simulink model "GBM1_2022b"  (R2022b)
settings: Solver=ode23t  StartTime=0  StopTime=130  FixedStep=0.005  MaxStep=0.005  RelTol=1e-3  EnableMultiTasking=on
values from neighbouring files (symbols this model uses):
  A1 = pi * 0.25^2    (= 0.196349540849)    [wecSimInputFile.m]
  A2 = pi * 0.01^2    (= 0.000314159265359)    [wecSimInputFile.m]
  C = 0.62    [wecSimInputFile.m]
  gDamping = 0    [wecSimInputFile.m]
  gStiffness = 0    [wecSimInputFile.m]
  rhoAir = 1.2    [wecSimInputFile.m]
  simu = simulationClass()    [wecSimInputFile.m]
  thresh = 0.3    [wecSimInputFile.m]
  waves = waveClass('irregular')    [wecSimInputFile.m]
undefined symbols (not defined in the file or in its folder): body, constraint, X, Y, Z
libraries: WECSim_Lib_Body_Elements x5, sm_lib x5, cstblocks x2, nesl_utility x2, vrlib x1, WECSim_Lib_Constraints x1, WECSim_Lib_Frames x1
(part 1 of 2)
settings Model: Creator=mlawson  LastModifiedBy=dforbus
settings SolverCC: ZeroCrossControl=DisableAll  AlgebraicLoopSolver=LineSearch  AutoInsertRateTranBlk=on
settings DataIOCC: SaveFormat=Array  SaveOutput=off  SaveTime=off  ReturnWorkspaceOutputs=off
settings OptimizationCC: LifeSpan=inf  SimCompilerOptimization=on
settings DebuggingCC: UnderspecifiedInitializationDetection=Classic  MergeDetectMultiDrivingBlocksExec=none  SolverPrmCheckMsg=warning  UnconnectedInputMsg=warning  UnconnectedOutputMsg=warning  UnconnectedLineMsg=warning  AllowSymbolicDim=off  StateNameClashWarn=warning  SFUnexpectedBacktrackingDiag=warning  SFNoUnconditionalDefaultTransitionDiag=warning  SFExecutionAtInitializationDiag=none  SFMachineParentedDataDiag=warning  ArithmeticOperatorsInVariantConditions=warning
settings HardwareCC: ProdBitPerPointer=32  ProdBitPerSizeT=32  ProdBitPerPtrDiffT=32  ProdLargestAtomicFloat=None  ProdIntDivRoundTo=Undefined  ProdEndianess=Unspecified  ProdWordSize=32  ProdHWDeviceType=32-bit Generic
settings ModelReferenceCC: EnableRefExpFcnMdlSchedulingChecks=on  PropagateSignalLabelsOutOfModel=off
settings SFSimCC: SimUseLocalCustomCode=off  CustomCodeUndefinedFunction=UseInterfaceOnly
settings RTWCC: RTWUseLocalCustomCode=off
settings CodeAppCC: StateflowObjectComments=on
settings GRTTargetCC: TargetLangStandard=C89/C90 (ANSI)
settings ConfigComp: CovMetricSettings=dw  CovSaveCumulativeToWorkspaceVar=on  CovSaveSingleToWorkspaceVar=on  CovExternalEMLEnable=off  CovSFcnEnable=off
settings SimscapeCC: SimscapeNormalizeSystem=off
settings ConfigurationSet: Description=SimMechanics 2G
settings ExplorerConfigSet: InternalSimMechanicsExplorerSettings="<ExplorerConfiguration><canonicalview>default</canonicalview><TilePanel><TileInfo><Tiles Columns=\"1\" Count=\"1\" Rows=\"1\"><Column Left=\"2\" Weight=\"1\"/><Column Left=\"1335\"/><Row Top=\"2\" Weight=\"1\"/><Row Top=\"911\"/><Tile Height=\"1\" Width=\"1\" X=\"0\" Y=\"0\"/></Tiles></TileInfo><SceneInfo><SceneViewer><BGColor><R>0.60000002384185791</R><G>0.60000002384185791</G><B>0.60000002384185791</B></BGColor><Camera><Position><X>365.37645888990272</X><Y>-369.82486814446582</Y><Z>359.64809521743916</Z></Position><Center><X>-6.7351450971904585</X><Y>2.2867358426280204</Y><Z>-12.463508769654169</Z></Center><Up><X>-0.40824829046386307</X><Y>0.40824829046386307</Y><Z>0.81649658092772615</Z></Up><Left>-57.820127362122818</Left><Right>57.820127362122818</Right><Bottom>-38.308817187253304</Bottom><Top>38.308817187253304</Top></Camera></SceneViewer></SceneInfo></TilePanel></ExplorerConfiguration>"

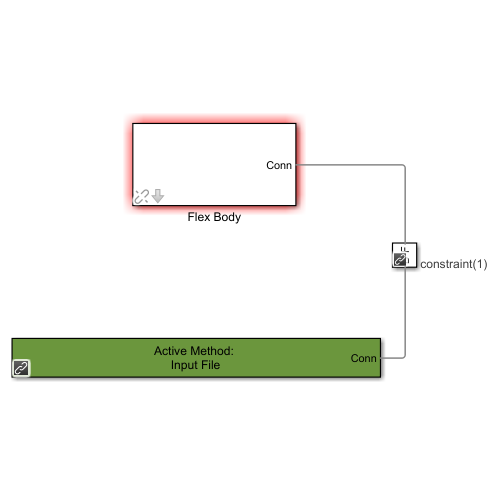
[thumbnail: Simulink's stored preview of the top-level diagram]
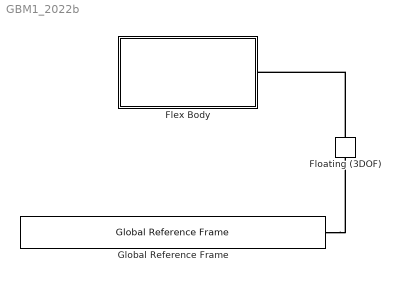
== system GBM1_2022b ==
  Flex Body : Subsystem  AncestorBlock=WECSim_Lib_Body_Elements/Flex Body  VariantControl=(default)  mask(Flex Body){body=body(1), InputFileText=Global Reference Frame option "Use Input File" is selected., h5File=hydroData/*.h5, geometryFile=geometry/*.stl, mass=0, inertia=0 0 0, nonHydro=0, nonlinearHydro=0, centerGravity=0 0 0, centerBuoyancy=0 0 0, dof=, volume=0, flex=1, displacement=0 0 0, axis=0 1 0, angle=0, option=0, cd=0 0 0, ca=0 0 0, area=0 0 0, VME=0, rgME=0 0 0, z=0 0 1}
      mask prompts: body "Body Number:"; mass "Body Mass [kg]:"; inertia "MoI [kg*m^2]:"; nonHydro "Nonhydro Body"; nonlinearHydro "Nonlinear Hydrodynamics"; centerGravity "Center of gravity [m]"; centerBuoyancy "Center of buoyancy [m]"; dof "Degrees of freedom"; volume "Displaced Volume [m^3]"; flex "Flexible Body"; displacement "Initial Linear Displacement"; axis "Initial Angular Displacement Axis"; angle "Initial Angular Displacement"; option "On/Off"; cd "Drag coefficient"; ca "Added mass coefficient"; area "Characteristic Area"; VME "Characteristic Volume"; rgME "Point of Application"; z "Z axis"
      mask help:
      | A Flex Body may contain generalized body modes that account for various bending, shear or other deformation modes. The BEM output must contain data for these additional DOFs.
      |
      | The variable name input below must be 'body(i)' where i=1,2,...
      | body(i) must be defined in the input file with the following fields:
      |
      |     .flexHydroBody = 1 (required)
      |             Float.
      |             Flag that creates a flex body. Set equal to 1 if the BEM data contains more than 6 degrees of freedom.
      |     .filename (required)
      |             String.
      |             The file path specifying the .h5 file for the body.
      |     .mass (required)
      |             Float or string.
      |             The translational interia or mass of the body in kg. If a string, the value must be 'equilibrium'. Default = [ ]
      |     .momOfIntertia (required)
      |             3x1 vector [Ixx Iyy Izz].
      |             Rotational intertia of the body in kg*m^2. Default = [ ]
      |     .geometryFile (optional)
      |             String
      |             Path to the geometry file of the body (.stl). Required for nonlinear hydrodynamics or visualization. Default = [ ]
      mask init:
      | if exist('body','var')
      |     % geometry file name
      |     h=[gcb '/Structure/Body Properties'];
      |     geomFile=body.geometryFile;
      |     set_param(h,'ExtGeomFileName',geomFile);
      |     geomType='STL';
      |     % split version e.g. '9.10.0.16028 (R2021a)' into 9, 10, 0, NaN.
      |     % cannot compare str2double('9.10') because it becomes '9.1' 
      |     ver=split(version,'.');
      |     ver=str2double(ver(1:3));
      |     if ver(1) < 9 || (ver(1) == 9 && ver(2) < 6)
      |        set_param(h,'ExtGeomFileType',geomType);
      |     end
      |     % toWorkSpace: outputs
      |     h=[gcb '/To Workspace'];
      |     responseName=['body' num2str(body.number) '_out'];
      |     set_param(h,'VariableName',responseName);
      |     % toWorkSpace: hydrostatic pressures
      |     h=[gcb '/Hydrostatic Restoring Force Calculation/Hydrostatic Restoring Force Calculation/Linear and Nonlinear Restoring Force Variant Subsystem/Nonlinear Hydrostatic Restoring Force/To Workspace1'];
      |     responseName=['body' num2str(body.number) '_hspressure_out'];
      |     set_param(h,'VariableName',responseName); 
      |     % toWorkSpace: wave pressures (nonlinear Froude-Krylov)
      |     h=[gcb '/Wave Diffraction and Excitation Force Calculation/Wave Diffraction and Excitation Force Calculation/Nonlinear FK Force Variant Subsystem/With Nonlinear FroudeKrylov Force/To Workspace'];
      |     responseName=['body' num2str(body.number) '_wavenonlinearpressure_out'];
      |     set_param(h,'VariableName',responseName);
      |     % toWorkSpace: wave pressures (linear Froude-Krylov)
      |     h=[gcb '/Wave Diffraction and Excitation Force Calculation/Wave Diffraction and Excitation Force Calculation/Nonlinear FK Force Variant Subsystem/With Nonlinear FroudeKrylov Force/To Workspace1'];
      |     responseName=['body' num2str(body.number) '_wavelinearpressure_out'];
      |     set_param(h,'VariableName',responseName);
      |     % position: GoTo 
      |     h=[gcb '/Goto'];
      |     responseName=['disp' num2str(body.number)];
      |     set_param(h,'GotoTag',responseName);
      |     % position: From
      |     h=[gcb '/From'];
      |     responseName=['disp' num2str(body.number)];
      |     set_param(h,'GotoTag',responseName);
      |     % velocity: GoTo 
      |     h=[gcb '/Goto1'];
      |     responseName=['vel' num2str(body.number)];
      |     set_param(h,'GotoTag',responseName);
      |     % velocity: From 
      |     h=[gcb '/From1'];
      |     responseName=['vel' num2str(body.number)];
      |     set_param(h,'GotoTag',responseName);
      |     % acceleration: GoTo 
      |     h=[gcb '/Goto2'];
      |     responseName=['acc' num2str(body.number)];
      |     set_param(h,'GotoTag',responseName);
      |     % acceleration: From 
      |     h=[gcb '/From2'];
      |     responseName=['acc' num2str(body.number)];
      |     set_param(h,'GotoTag',responseName);
      |     %%
      |     % Flex Body Morison Element: Off
      |     h = [gcb '/Morrison Element and Viscous Damping Force Calculation/Morison Element and Viscous Damping Force Calculation/Morison Element Variant Subsystem/Morison Element Off'];
      |     responseName = ['sv_b' num2str(body.number) '_MEOff'];
      |     set_param(h,'VariantControl',responseName);
      |     %%
      |     % Flex Body Morison Element: On
      |     h = [gcb '/Morrison Element and Viscous Damping Force Calculation/Morison Element and Viscous Damping Force Calculation/Morison Element Variant Subsystem/Morison Element On'];
      |     responseName = ['sv_b' num2str(body.number) '_MEOn'];
      |     set_param(h,'VariantControl',responseName);
      |     %%
      |     % Flex Body Nonlinear FroudeKrylov Force: Off
      |     h = [gcb '/Wave Diffraction and Excitation Force Calculation/Wave Diffraction and Excitation Force Calculation/Nonlinear FK Force Variant Subsystem/No Nonlinear FroudeKrylov Force'];
      |     responseName = ['sv_b' num2str(body.number) '_linearHydro'];
      |     set_param(h,'VariantControl',responseName);
      |     %%
      |     % Flex Body Nonlinear FroudeKrylov Force: On
      |     h = [gcb '/Wave Diffraction and Excitation Force Calculation/Wave Diffraction and Excitation Force Calculation/Nonlinear FK Force Variant Subsystem/With Nonlinear FroudeKrylov Force'];
      |     responseName = ['sv_b' num2str(body.number) '_nonlinearHydro'];
      |     set_param(h,'VariantControl',responseName);
      |     %%
      |     % Flex Body Nonlinear Restoring: Off
      |     h = [gcb '/Hydrostatic Restoring Force Calculation/Hydrostatic Restoring Force Calculation/Linear and Nonlinear Restoring Force Variant Subsystem/Linear Hydrostatic Restoring Force'];
      |     responseName = ['sv_b' num2str(body.number) '_linearHydro'];
      |     set_param(h,'VariantControl',responseName);
      |     %%
      |     % Flex Body Nonlinear Restoring: On
      |     h = [gcb '/Hydrostatic Restoring Force Calculation/Hydrostatic Restoring Force Calculation/Linear and Nonlinear Restoring Force Variant Subsystem/Nonlinear Hydrostatic Restoring Force'];
      |     responseName = ['sv_b' num2str(body.number) '_nonlinearHydro'];
      |     set_param(h,'VariantControl',responseName);
      |     %%
      |     % Flex Body Nonlinear FroudeKrylov or Restoring: Instantaneous Free Surface
      |     h = [gcb '/Nonlinear Wave Elevation/Linear or Instantaneous Free Surface/Instantaneous Water Free Surface'];
      |     responseName = ['sv_b' num2str(body.number) '_instFS'];
      |     set_param(h,'VariantControl',responseName);
      |     %%
      |     % Flex Body Nonlinear FroudeKrylov or Restoring: Mean Free Surface
      |     h = [gcb '/Nonlinear Wave Elevation/Linear or Instantaneous Free Surface/Mean Water Free Surface'];
      |     responseName = ['sv_b' num2str(body.number) '_meanFS'];
      |     set_param(h,'VariantControl',responseName);
      |     %%
      | end
      settings: LibrarySourceBlock=WECSim_Lib_Body_Elements/Flex Body
      mask Help:
      | A Flex Body may contain generalized body modes that account for various bending, shear or other deformation modes. The BEM output must contain data for these additional DOFs.
      | 
      | The variable name input below must be 'body(i)' where i=1,2,...
      | body(i) must be defined in the input file with the following fields:
      | 
      |     .flexHydroBody = 1 (required)
      |             Float.
      |             Flag that creates a flex body. Set equal to 1 if the BEM data contains more than 6 degrees of freedom.
      |     .filename (required)
      |             String.
      |             The file path specifying the .h5 file for the body.
      |     .mass (required)
      |             Float or string.
      |             The translational interia or mass of the body in kg. If a string, the value must be 'equilibrium'. Default = [ ]
      |     .momOfIntertia (required)
      |             3x1 vector [Ixx Iyy Izz].
      |             Rotational intertia of the body in kg*m^2. Default = [ ]
      |     .geometryFile (optional)
      |             String
      |             Path to the geometry file of the body (.stl). Required for nonlinear hydrodynamics or visualization. Default = [ ]
      mask TypeOptions nonHydro: 0 | 1 | 2
      mask Callback nonHydro: bodyClassCallback(gcbh)
      mask TypeOptions nonlinearHydro: 0 | 1 | 2
      mask TypeOptions flex: 0 | 1
      mask TypeOptions option: 0 | 1 | 2
      mask Callback option: bodyClassCallback(gcbh)
      mask DialogControl CustomParameterGroup Prompt: Custom Parameters
      mask DialogControl std_opts Prompt: Standard Options
      mask DialogControl H5button Prompt: Select .h5 File
      mask DialogControl H5button Callback: h5ButtonCallback(gcbh)
      mask DialogControl STLbutton Prompt: Select .stl File
      mask DialogControl STLbutton Callback: stlButtonCallback(gcbh)
      mask DialogControl inertia Tooltip: Moment of Inertia
      mask DialogControl initial Prompt: Initial Displacement
      mask DialogControl morisonElement Prompt: Morison Element
      mask DialogControl rgME Tooltip: The vector from the body COG to point of application for the Morison Element
      mask DialogControl z Tooltip: The unit normal vector center axis of the Morison Element
  Floating (3DOF) : WECSim_Lib_Constraints/Floating (3DOF)  constraint=constraint(1)  loc="0  0  0"  displacement=0 0 0  y=0 1 0  z=0 0 1  upperLimitSpecify=off  upperLimitBound=0  upperLimitTransitionRegionWidth=0  upperLimitStiffness=0  upperLimitDamping=0  lowerLimitSpecify=off  lowerLimitBound=0  lowerLimitTransitionRegionWidth=0  lowerLimitStiffness=0  lowerLimitDamping=0
      settings: AttributesFormatString=%<constraint>
  Global Reference Frame : WECSim_Lib_Frames/Global Reference Frame  waves=waves  simu=simu  InputMethod=Input File  InputFile=wecSimInputFile.m  mode=normal  explorer=off  solver=ode4  startTime=0  rampTime=100  endTime=400  dt=0.1  cicEndTime=60  stateSpace=0  WaveClass=regular  height=2.5  period=8  elevationFile=NOT DEFINED  spectrumFile=NOT DEFINED  direction=0  spread=1  spectrumType=NOT DEFINED  phaseSeed=0  option=EqualEnergy
  connections:
  Global Reference Frame/RConn1 -- Floating (3DOF)/LConn1
  Floating (3DOF)/RConn1 -- Flex Body/RConn1

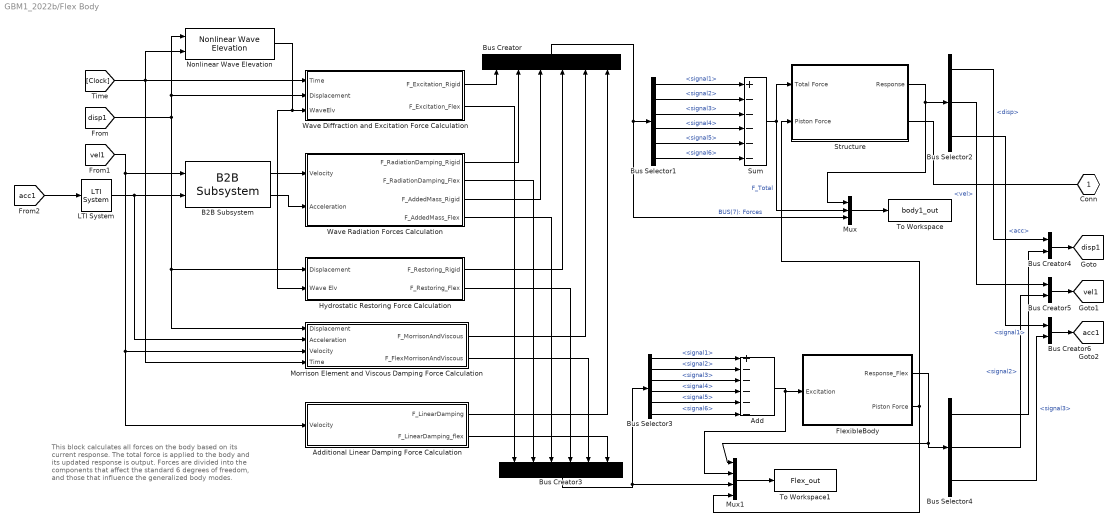
== system GBM1_2022b/Flex Body ==
  note: This block calculates all forces on the body based on its current response. The total force is applied to the body and its updated response is output.
      |
      | Forces are divided into the components that affect the standard 6 degrees of freedom, and those that influence the generalized body modes.
  Add : Sum  Inputs=+-----
  Additional Linear Damping Force Calculation : Subsystem
  B2B Subsystem : WECSim_Lib_Body_Elements/Rigid Body/Hydrodynamic Body/B2B Subsystem  SystemSampleTime=-1  VariantActivationTime=update diagram  Latency=0  AutoFrameSizeCalculation=off
  Bus Creator : BusCreator  Inputs=6
  Bus Creator3 : BusCreator  Inputs=6
  Bus Creator4 : BusCreator  Inputs=2
  Bus Creator5 : BusCreator  Inputs=2
  Bus Creator6 : BusCreator  Inputs=2
  Bus Selector1 : BusSelector  OutputSignals=signal1,signal2,signal3,signal4,signal5,signal6
  Bus Selector2 : BusSelector  OutputSignals=disp,vel,acc
  Bus Selector3 : BusSelector  OutputSignals=signal1,signal2,signal3,signal4,signal5,signal6
  Bus Selector4 : BusSelector  OutputSignals=signal1,signal2,signal3
  FlexibleBody : Subsystem
  Hydrostatic Restoring Force Calculation : Subsystem
  LTI System : cstblocks/LTI System  sys=LPF50  IC=[]
  Morrison Element and Viscous Damping Force Calculation : Subsystem
  Mux : Mux  Inputs=3
  Mux1 : Mux
  Nonlinear Wave Elevation : WECSim_Lib_Body_Elements/Rigid Body/Hydrodynamic Body/Nonlinear Wave Elevation  SystemSampleTime=simu.nonlinearDt  VariantActivationTime=update diagram  Latency=0  AutoFrameSizeCalculation=off
  Structure : Subsystem
  Sum : Sum  Inputs=+-----
  To Workspace : ToWorkspace  VariableName=body1_out  SaveFormat=Structure With Time  SampleTime=simu.dtOut
  To Workspace1 : ToWorkspace  VariableName=Flex_out  SaveFormat=Structure With Time  SampleTime=simu.dtOut
  Wave Diffraction and Excitation Force Calculation : Subsystem
  Wave Radiation Forces Calculation : Subsystem
  Conn : PMIOPort  Side=Right
  tag scope: acc1=global, disp1=global, vel1=global
  wires:
  LTI System/1 -> Morrison Element and Viscous Damping Force Calculation/2(Acceleration), B2B Subsystem/2
  [acc1] -> LTI System/1
  Morrison Element and Viscous Damping Force Calculation/1(F_MorrisonAndViscous) -> Bus Creator/5
  Hydrostatic Restoring Force Calculation/2(F_Restoring_Flex) -> Bus Creator3/4
  Bus Selector2/3 -> Bus Creator6/1  "<acc>"
  Bus Selector2/2 -> Bus Creator5/1  "<vel>"
  Bus Creator6/1 -> [acc1]
  Bus Creator5/1 -> [vel1]
  Bus Creator4/1 -> [disp1]
  Bus Selector2/1 -> Bus Creator4/1  "<disp>"
  Bus Selector3/6 -> Add/6  "<signal6>"
  Additional Linear Damping Force Calculation/2(F_LinearDamping_flex) -> Bus Creator3/6
  Bus Selector3/5 -> Add/5  "<signal5>"
  Morrison Element and Viscous Damping Force Calculation/2("F_FlexMorrisonAndViscous ") -> Bus Creator3/5
  Additional Linear Damping Force Calculation/1(F_LinearDamping) -> Bus Creator/6
  Bus Selector4/3 -> Bus Creator6/2  "<signal3>"
  Bus Selector4/2 -> Bus Creator5/2  "<signal2>"
  Bus Selector4/1 -> Bus Creator4/2  "<signal1>"
  FlexibleBody/1(Response_Flex) -> Mux1/1, Bus Selector4/1
  Add/1 -> FlexibleBody/1(Excitation), Mux1/2
  Bus Selector3/4 -> Add/4  "<signal4>"
  Bus Selector3/3 -> Add/3  "<signal3>"
  Bus Selector3/2 -> Add/2  "<signal2>"
  Bus Selector3/1 -> Add/1  "<signal1>"
  Bus Creator3/1 -> Mux1/3, Bus Selector3/1
  Wave Radiation Forces Calculation/4(F_AddedMass_Flex) -> Bus Creator3/3
  Wave Radiation Forces Calculation/2(F_RadiationDamping_Flex) -> Bus Creator3/2
  Wave Diffraction and Excitation Force Calculation/2(F_Excitation_Flex) -> Bus Creator3/1
  Mux1/1 -> To Workspace1/1
  [Clock] -> Wave Diffraction and Excitation Force Calculation/1(Time), Morrison Element and Viscous Damping Force Calculation/4(Time), Nonlinear Wave Elevation/2
  Wave Radiation Forces Calculation/3(F_AddedMass_Rigid) -> Bus Creator/3
  Wave Diffraction and Excitation Force Calculation/1(F_Excitation_Rigid) -> Bus Creator/1
  Wave Radiation Forces Calculation/1(F_RadiationDamping_Rigid) -> Bus Creator/2
  Hydrostatic Restoring Force Calculation/1(F_Restoring_Rigid) -> Bus Creator/4
  Nonlinear Wave Elevation/1 -> Wave Diffraction and Excitation Force Calculation/3(WaveElv), Hydrostatic Restoring Force Calculation/2(Wave Elv)
  [disp1] -> Hydrostatic Restoring Force Calculation/1(Displacement), Morrison Element and Viscous Damping Force Calculation/1(Displacement), Wave Diffraction and Excitation Force Calculation/2(Displacement), Nonlinear Wave Elevation/1
  B2B Subsystem/1 -> Wave Radiation Forces Calculation/1(Velocity)
  B2B Subsystem/2 -> Wave Radiation Forces Calculation/2(Acceleration)
  [vel1] -> B2B Subsystem/1, Morrison Element and Viscous Damping Force Calculation/3(Velocity), Additional Linear Damping Force Calculation/1(Velocity)
  Bus Selector1/6 -> Sum/6  "<signal6>"
  Bus Selector1/1 -> Sum/1  "<signal1>"
  Bus Selector1/2 -> Sum/2  "<signal2>"
  Bus Selector1/5 -> Sum/5  "<signal5>"
  Bus Selector1/3 -> Sum/3  "<signal3>"
  Bus Selector1/4 -> Sum/4  "<signal4>"
  Mux/1 -> To Workspace/1
  Sum/1 -> Structure/1(Total Force), Mux/2  "F_Total"
  Structure/1(Response) -> Bus Selector2/1, Mux/1
  Bus Creator/1 -> Bus Selector1/1, Mux/3  "BUS(7): Forces"
  FlexibleBody/2(Piston Force) -> Structure/2(Piston Force), Mux1/4
  connections:
  Conn/RConn1 -- Structure/RConn1

== system GBM1_2022b/Flex Body/Additional Linear Damping Force Calculation ==
  Velocity : Inport
  Additional Linear Damping Force Calculation : WECSim_Lib_Body_Elements/Rigid Body/Hydrodynamic Body/Additional Linear Damping Force Calculation  SystemSampleTime=-1  VariantActivationTime=update diagram  Latency=0  AutoFrameSizeCalculation=off
  Selector : Selector  InputPortWidth=body.dof  IndexOptions=Index vector (dialog)  Indices=[1:6]  OutputSizes=1
  Selector1 : Selector  InputPortWidth=body.dof  IndexOptions=Index vector (dialog)  Indices=[7:body.dofEnd]  OutputSizes=1
  F_LinearDamping : Outport  PortDimensions=6
  F_LinearDamping_flex : Outport  Port=2  PortDimensions=body.gbmDOF
  wires:
  Additional Linear Damping Force Calculation/1 -> Selector1/1, Selector/1
  Velocity/1 -> Additional Linear Damping Force Calculation/1  "v"
  Selector1/1 -> F_LinearDamping_flex/1
  Selector/1 -> F_LinearDamping/1

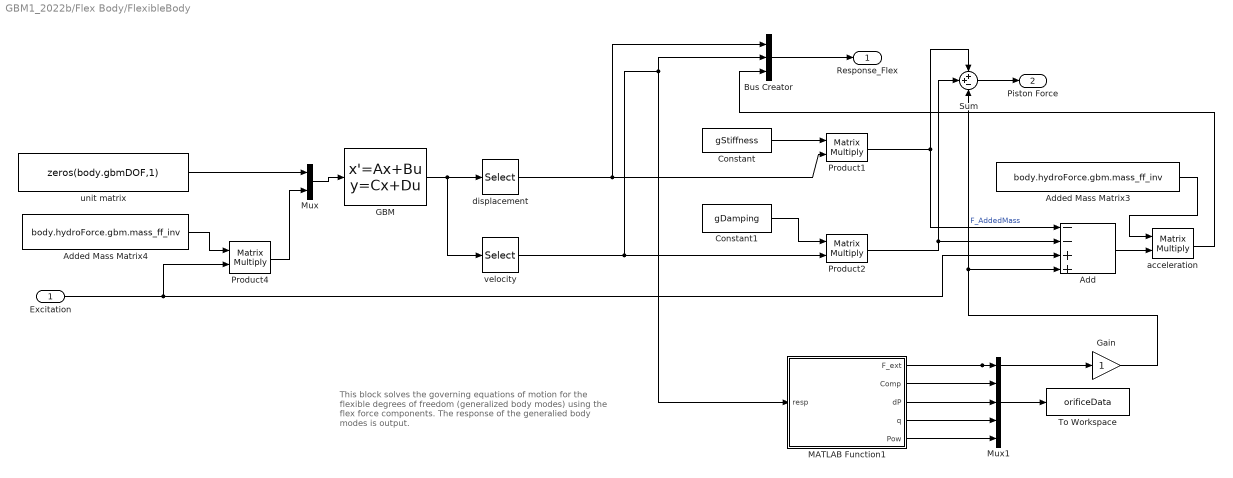
== system GBM1_2022b/Flex Body/FlexibleBody ==
  note: This block solves the governing equations of motion for the flexible degrees of freedom (generalized body modes) using the flex force components. The response of the generalied body modes is output.
  Excitation : Inport
  Add : Sum  Inputs=--++
  Added Mass Matrix3 : Constant  Value=body.hydroForce.gbm.mass_ff_inv
  Added Mass Matrix4 : Constant  Value=body.hydroForce.gbm.mass_ff_inv
  Bus Creator : BusCreator  Inputs=3
  Constant : Constant  Value=gStiffness
  Constant1 : Constant  Value=gDamping
  GBM : StateSpace  A=body.hydroForce.gbm.state_space.A  B=body.hydroForce.gbm.state_space.B  C=body.hydroForce.gbm.state_space.C  D=body.hydroForce.gbm.state_space.D  InitialCondition=0
  Gain : Gain
  MATLAB Function1 : MATLAB Function  TreatAsAtomicUnit=on
  Mux : Mux  Inputs=2
  Mux1 : Mux  Inputs=5
  Product1 : Product  Multiplication=Matrix(*)
  Product2 : Product  Multiplication=Matrix(*)
  Product4 : Product  Multiplication=Matrix(*)
  Sum : Sum  Inputs=++-
  To Workspace : ToWorkspace  VariableName=orificeData  SaveFormat=Structure With Time  SampleTime=-1
  acceleration : Product  Multiplication=Matrix(*)
  displacement : Selector  InputPortWidth=body.gbmDOF*2  IndexOptions=Index vector (dialog)  Indices=[1:body.gbmDOF]  OutputSizes=1
  unit matrix : Constant  Value=zeros(body.gbmDOF,1)
  velocity : Selector  InputPortWidth=2*body.gbmDOF  IndexOptions=Index vector (dialog)  Indices=[body.gbmDOF+1:2*body.gbmDOF]  OutputSizes=1
  Response_Flex : Outport
  Piston Force : Outport  Port=2
  wires:
  acceleration/1 -> Bus Creator/3
  Bus Creator/1 -> Response_Flex/1
  Mux/1 -> GBM/1
  Product4/1 -> Mux/2
  Added Mass Matrix4/1 -> Product4/1
  unit matrix/1 -> Mux/1
  Add/1 -> acceleration/2
  Added Mass Matrix3/1 -> acceleration/1
  Product1/1 -> Add/1, Sum/1  "F_AddedMass"
  Constant1/1 -> Product2/1
  Constant/1 -> Product1/1
  GBM/1 -> velocity/1, displacement/1
  Product2/1 -> Sum/2, Add/2
  Sum/1 -> Piston Force/1
  MATLAB Function1/1(F_ext) -> Mux1/1, Gain/1
  Mux1/1 -> To Workspace/1
  MATLAB Function1/2(Comp) -> Mux1/2
  MATLAB Function1/3(dP) -> Mux1/3
  MATLAB Function1/4(q) -> Mux1/4
  MATLAB Function1/5(Pow) -> Mux1/5
  velocity/1 -> MATLAB Function1/1(resp), Bus Creator/2, Product2/2
  displacement/1 -> Bus Creator/1, Product1/2
  Excitation/1 -> Add/3, Product4/2
  Gain/1 -> Add/4, Sum/3

== system GBM1_2022b/Flex Body/Hydrostatic Restoring Force Calculation ==
  note: Do not link the `Hydrostatic Restoring Force Calculation`
      | to the rigid body block, this will break the Flex Body block.
  Displacement : Inport
  Wave Elv : Inport  Port=2
  Hydrostatic Restoring Force Calculation : Subsystem
  Selector : Selector  InputPortWidth=body.dof  IndexOptions=Index vector (dialog)  Indices=[1:6]  OutputSizes=1
  Selector1 : Selector  InputPortWidth=body.dof  IndexOptions=Index vector (dialog)  Indices=[7:body.dofEnd]  OutputSizes=1
  F_Restoring_Rigid : Outport  PortDimensions=6
  F_Restoring_Flex : Outport  Port=2  PortDimensions=body.gbmDOF
  wires:
  Wave Elv/1 -> Hydrostatic Restoring Force Calculation/2(Wave Elv)
  Displacement/1 -> Hydrostatic Restoring Force Calculation/1(Displacement)  "x"
  Selector1/1 -> F_Restoring_Flex/1
  Selector/1 -> F_Restoring_Rigid/1
  Hydrostatic Restoring Force Calculation/1(F_Restoring) -> Selector/1, Selector1/1  "F_Restoring"

== system GBM1_2022b/Flex Body/Morrison Element and Viscous Damping Force Calculation ==
  Displacement : Inport
  Acceleration : Inport  Port=2
  Velocity : Inport  Port=3
  Time : Inport  Port=4
  Morison Element and Viscous Damping Force Calculation : Subsystem  AncestorBlock=WECSim_Lib_Body_Elements/Rigid Body/Hydrodynamic Body/Morison Element and Viscous Damping Force Calculation
      settings: LibrarySourceBlock=WECSim_Lib_Body_Elements/Rigid Body/Hydrodynamic Body/Morison Element and Viscous Damping Force Calculation
  Selector : Selector  InputPortWidth=body.dof  IndexOptions=Index vector (dialog)  Indices=[1:6]  OutputSizes=1
  Selector1 : Selector  InputPortWidth=body.dof  IndexOptions=Index vector (dialog)  Indices=[7:body.dofEnd]  OutputSizes=1
  F_MorrisonAndViscous : Outport  PortDimensions=6
  "F_FlexMorrisonAndViscous " : Outport  Port=2  PortDimensions=body.gbmDOF
  wires:
  Selector1/1 -> "F_FlexMorrisonAndViscous "/1
  Selector/1 -> F_MorrisonAndViscous/1
  Morison Element and Viscous Damping Force Calculation/1(F_MorisonAndViscous) -> Selector/1, Selector1/1
  Velocity/1 -> Morison Element and Viscous Damping Force Calculation/3(Velocity)
  Displacement/1 -> Morison Element and Viscous Damping Force Calculation/1(Displacement)
  Time/1 -> Morison Element and Viscous Damping Force Calculation/4(Time)
  Acceleration/1 -> Morison Element and Viscous Damping Force Calculation/2(Acceleration)

== system GBM1_2022b/Flex Body/Structure ==
  note: Apply the total force to the body and calculate its response relative to the global reference frame.
      |
      | Output force to apply to another body.
  Total Force : Inport
  Piston Force : Inport  Port=2
  Body Properties : sm_lib/Body Elements/File Solid  ExtGeomFileName=../geometry/float.stl  UnitType=Custom  ExtGeomFileUnits=m  StepReaderType=HEX  ExportConvexHullGeometry=off  InertiaType=Custom  Mass=body.mass  MassUnits=kg  CenterOfMass=[0 0 0]  CenterOfMassUnits=m  MomentsOfInertia=body.inertia  MomentsOfInertiaUnits=kg*m^2  ProductsOfInertia=[0 0 0]  ProductsOfInertiaUnits=kg*m^2  BasedOnType=Density  Density=1000  DensityUnits=kg/(m^3)  DoExposeReferenceFrame=on  SerializedFrames=<Frames/>  GraphicType=FromGeometry  MarkerShape=Sphere  MarkerSize=10  MarkerSizeUnits=m  GraphicVisPropType=SimpleVisualProperties  GraphicDiffuseColor=body.viz.color  GraphicSpecularColor=[0.5 0.5 0.5 1.0]  GraphicAmbientColor=[0.15 0.15 0.15 1.0]  GraphicEmissiveColor=[0.0 0.0 0.0 1.0]  GraphicShininess=75  GraphicOpacity=body.viz.opacity
  Demux : Demux  Outputs=3
  External Force and Torque : sm_lib/Forces and Torques/External Force and Torque  ForceResolutionFrame=World  EnableForceX=off  EnableForceY=off  EnableForceZ=off  EnableForce=on  TorqueResolutionFrame=World  EnableTorqueX=off  EnableTorqueY=off  EnableTorqueZ=off  EnableTorque=on
  Motion Sensor : WECSim_Lib_Body_Elements/Rigid Body/Hydrodynamic Body/Structure/Motion Sensor  SystemSampleTime=-1  VariantActivationTime=update diagram  Latency=0  AutoFrameSizeCalculation=off
  Mux : Mux  Inputs=3
  Rigid Transform (Setup CG) : sm_lib/Frames and Transforms/Rigid Transform  TranslationMethod=Cartesian  TranslationStandardOffset=0  TranslationLengthUnit=m  TranslationStandardAxis=+Z  TranslationCartesianOffset=body.centerGravity  TranslationROffset=0  TranslationROffsetUnits=m  TranslationZOffset=0  TranslationZOffsetUnits=m  TranslationThetaOffset=0  TranslationThetaOffsetUnits=deg  RotationMethod=None  RotationAngleUnits=rad  RotationStandardAxis=+Y  RotationAngle=0.05  RotationArbitraryAxis=[0.57735026918962584 0.57735026918962584 0.57735026918962584]  FollAlignAxisA=+X  BaseAlignAxisA=+Y  FollAlignAxisB=+Y  BaseAlignAxisB=+Z  RotationSequenceAxes=FollowerAxes  RotationSequence=XYX  RotationSequenceAngles=[0 0 0]  RotationSequenceAnglesUnits=deg  RotationMatrix=[1 0 0; 0 1 0; 0 0 1]  Quaternion=[1 0 0 0]
  Rigid Transform (Setup Initial Disp) : sm_lib/Frames and Transforms/Rigid Transform  TranslationMethod=Cartesian  TranslationStandardOffset=0  TranslationLengthUnit=m  TranslationStandardAxis=+Z  TranslationCartesianOffset=body.initial.displacement  TranslationROffset=0  TranslationROffsetUnits=m  TranslationZOffset=0  TranslationZOffsetUnits=m  TranslationThetaOffset=0  TranslationThetaOffsetUnits=deg  RotationMethod=ArbitraryAxis  RotationAngleUnits=rad  RotationStandardAxis=+Y  RotationAngle=body.initial.angle  RotationArbitraryAxis=body.initial.axis  FollAlignAxisA=+X  BaseAlignAxisA=+Y  FollAlignAxisB=+Y  BaseAlignAxisB=+Z  RotationSequenceAxes=FollowerAxes  RotationSequence=XYX  RotationSequenceAngles=[0 0 0]  RotationSequenceAnglesUnits=deg  RotationMatrix=[1 0 0; 0 1 0; 0 0 1]  Quaternion=[1 0 0 0]
  Selector : Selector  InputPortWidth=6  IndexOptions=Index vector (dialog)  Indices=[1:3]  OutputSizes=1
  Selector1 : Selector  InputPortWidth=6  IndexOptions=Index vector (dialog)  Indices=[4:6]  OutputSizes=1
  Simulink-PS Converter1 : nesl_utility/Simulink-PS Converter  PhysicalDomain=network_engine_domain  SubClassName=ps_input  LeftPortType=input  RightPortType=output  PseudoPeriodic=off  Frequencies=[]  NoiseDistribution=none  NoiseParameters=[]  Unit=1  AffineConversion=off  FilteringAndDerivatives=zero  SimscapeFilterOrder=1  InputFilterTimeConstant=0.001  UdotUserProvided=1
  Simulink-PS Converter2 : nesl_utility/Simulink-PS Converter  PhysicalDomain=network_engine_domain  SubClassName=ps_input  LeftPortType=input  RightPortType=output  PseudoPeriodic=off  Frequencies=[]  NoiseDistribution=none  NoiseParameters=[]  Unit=1  AffineConversion=off  FilteringAndDerivatives=zero  SimscapeFilterOrder=1  InputFilterTimeConstant=0.001  UdotUserProvided=1
  Sum : Sum  Inputs=++|
  World Frame : sm_lib/Frames and Transforms/World Frame
  Conn Free Surface : PMIOPort  Side=Right
  Response : Outport
  wires:
  Motion Sensor/1 -> Response/1
  Selector1/1 -> Simulink-PS Converter2/1
  Total Force/1 -> Selector/1, Selector1/1
  Selector/1 -> Demux/1
  Mux/1 -> Simulink-PS Converter1/1
  Demux/3 -> Sum/2
  Sum/1 -> Mux/3
  Piston Force/1 -> Sum/1
  Demux/2 -> Mux/2
  Demux/1 -> Mux/1
  connections:
  Motion Sensor/LConn1 -- World Frame/RConn1
  Rigid Transform (Setup Initial Disp)/LConn1 -- Rigid Transform (Setup CG)/RConn1
  Conn Free Surface/RConn1 -- Rigid Transform (Setup CG)/LConn1
  Motion Sensor/RConn1 -- Body Properties/RConn1 -- Rigid Transform (Setup Initial Disp)/RConn1 -- External Force and Torque/RConn1
  External Force and Torque/LConn2 -- Simulink-PS Converter2/RConn1
  External Force and Torque/LConn1 -- Simulink-PS Converter1/RConn1

== system GBM1_2022b/Flex Body/Wave Diffraction and Excitation Force Calculation ==
  note: Do not link the `Wave Diffraction and Excitation Force Calculation`
      | to the rigid body block, this will break the Flex Body block.
  Time : Inport
  Displacement : Inport  Port=2
  WaveElv : Inport  Port=3
  Selector : Selector  InputPortWidth=body.dof  IndexOptions=Index vector (dialog)  Indices=[1:6]  OutputSizes=1
  Selector1 : Selector  InputPortWidth=body.dof  IndexOptions=Index vector (dialog)  Indices=[7:body.dofEnd]  OutputSizes=1
  Wave Diffraction and Excitation Force Calculation : Subsystem
  F_Excitation_Rigid : Outport  PortDimensions=6
  F_Excitation_Flex : Outport  Port=2  PortDimensions=body.gbmDOF
  wires:
  Displacement/1 -> Wave Diffraction and Excitation Force Calculation/2(Displacement)
  WaveElv/1 -> Wave Diffraction and Excitation Force Calculation/3(WaveElv)
  Time/1 -> Wave Diffraction and Excitation Force Calculation/1(Time)
  Selector1/1 -> F_Excitation_Flex/1
  Selector/1 -> F_Excitation_Rigid/1
  Wave Diffraction and Excitation Force Calculation/1(F_Excitation) -> Selector/1, Selector1/1

== system GBM1_2022b/Flex Body/Wave Radiation Forces Calculation ==
  Velocity : Inport
  Acceleration : Inport  Port=2
  Selector : Selector  InputPortWidth=body.dof  IndexOptions=Index vector (dialog)  Indices=[1:6]  OutputSizes=1
  Selector1 : Selector  InputPortWidth=body.dof  IndexOptions=Index vector (dialog)  Indices=[7:body.dofEnd]  OutputSizes=1
  Selector2 : Selector  InputPortWidth=body.dof  IndexOptions=Index vector (dialog)  Indices=[1:6]  OutputSizes=1
  Selector3 : Selector  InputPortWidth=body.dof  IndexOptions=Index vector (dialog)  Indices=[7:body.dofEnd]  OutputSizes=1
  Wave Radiation Forces Calculation : WECSim_Lib_Body_Elements/Rigid Body/Hydrodynamic Body/Wave Radiation Forces Calculation  SystemSampleTime=-1  VariantActivationTime=update diagram  Latency=0  AutoFrameSizeCalculation=off
  F_RadiationDamping_Rigid : Outport  PortDimensions=6
  F_RadiationDamping_Flex : Outport  Port=2  PortDimensions=body.gbmDOF
  F_AddedMass_Rigid : Outport  Port=3  PortDimensions=6
  F_AddedMass_Flex : Outport  Port=4  PortDimensions=body.gbmDOF
  wires:
  Velocity/1 -> Wave Radiation Forces Calculation/1
  Acceleration/1 -> Wave Radiation Forces Calculation/2
  Wave Radiation Forces Calculation/1 -> Selector1/1, Selector/1  "F_RadiationDamping"
  Selector1/1 -> F_RadiationDamping_Flex/1
  Selector/1 -> F_RadiationDamping_Rigid/1
  Selector3/1 -> F_AddedMass_Flex/1
  Selector2/1 -> F_AddedMass_Rigid/1
  Wave Radiation Forces Calculation/2 -> Selector2/1, Selector3/1  "F_AddedMass"

== system GBM1_2022b/Flex Body/Hydrostatic Restoring Force Calculation/Hydrostatic Restoring Force Calculation ==
  Displacement : Inport
  Wave Elv : Inport  Port=2
  Add : Sum  Inputs=+-
  Center of Gravity : Constant  Value=body.centerGravity
  Constant : Constant  Value=zeros(1,body.dof-3)
  Linear and Nonlinear Restoring Force Variant Subsystem : Subsystem  Variant=on
  Mux : Mux  Inputs=2
  F_Restoring : Outport
  wires:
  Displacement/1 -> Add/1  "x"
  Linear and Nonlinear Restoring Force Variant Subsystem/1(Out1) -> F_Restoring/1  "F_Restoring"
  Mux/1 -> Add/2
  Center of Gravity/1 -> Mux/1  "cg"
  Constant/1 -> Mux/2
  Wave Elv/1 -> Linear and Nonlinear Restoring Force Variant Subsystem/2(In2)
  Add/1 -> Linear and Nonlinear Restoring Force Variant Subsystem/1(In1)  "x_cg"

== system GBM1_2022b/Flex Body/Morrison Element and Viscous Damping Force Calculation/Morison Element and Viscous Damping Force Calculation ==
  note: The output force is a combination of the quadratic viscous drag force and the Morison element force.
      |
      | F_quadraticViscous = 0.5*Cd*rho*A*v*|v|
  Displacement : Inport
  Acceleration : Inport  Port=2
  Velocity : Inport  Port=3
  Time : Inport  Port=4
  Abs1 : Abs  SaturateOnIntegerOverflow=off
  LTI System : cstblocks/LTI System  sys=LPF50  IC=[]
  Morison Element Variant Subsystem : Subsystem  Variant=on
  Product : Product
  Product1 : Product  Multiplication=Matrix(*)
  "VisSum " : Sum  Inputs=+-
  "Viscous Damping Matrix (diagonal) " : Constant  Value=body.hydroForce.quadDrag
  F_MorisonAndViscous : Outport
  wires:
  Morison Element Variant Subsystem/1(morison_force) -> "VisSum "/2
  Velocity/1 -> Abs1/1, Morison Element Variant Subsystem/2(velocity), Product/1
  LTI System/1 -> Morison Element Variant Subsystem/3(acceleration)
  Displacement/1 -> Morison Element Variant Subsystem/1(displacement)
  Time/1 -> Morison Element Variant Subsystem/4(time)
  Product/1 -> Product1/2  "v * |v|"
  "Viscous Damping Matrix (diagonal) "/1 -> Product1/1  "0.5 * cd * rho *A"
  Product1/1 -> "VisSum "/1  "F_quadraticViscous"
  Abs1/1 -> Product/2
  Acceleration/1 -> LTI System/1
  "VisSum "/1 -> F_MorisonAndViscous/1  "F_MorisonAndViscous"

== system GBM1_2022b/Flex Body/Wave Diffraction and Excitation Force Calculation/Wave Diffraction and Excitation Force Calculation ==
  note: The excitation force = F_wave * ramp function
  Time : Inport
  Displacement : Inport  Port=2
  WaveElv : Inport  Port=3
  Add : Sum
  Constant : Constant
  Less Than : RelationalOperator  Operator=<  OutDataTypeStr=boolean  RndMeth=Simplest  InputSameDT=off
  Linear Wave Excitation Force Variant Subsystem : Subsystem  Variant=on
  Nonlinear FK Force Variant Subsystem : Subsystem  Variant=on
  Product : Product
  Ramp Function Time : Constant  Value=simu.rampTime
  Ramp function : Subsystem
  Switch : Switch  Criteria=u2 ~= 0  SaturateOnIntegerOverflow=off  InputSameDT=off
  F_Excitation : Outport  PortDimensions=body.dof
  wires:
  Ramp Function Time/1 -> Less Than/2
  Constant/1 -> Switch/3
  Time/1 -> Ramp function/1(Time), Less Than/1, Linear Wave Excitation Force Variant Subsystem/1(Time), Nonlinear FK Force Variant Subsystem/1(Time)
  Ramp function/1(R) -> Switch/1
  Less Than/1 -> Switch/2
  Nonlinear FK Force Variant Subsystem/1(Nonlinear Excitation) -> Add/2
  Linear Wave Excitation Force Variant Subsystem/1(Linear Excitation) -> Add/1
  WaveElv/1 -> Nonlinear FK Force Variant Subsystem/3(WaveElv)
  Displacement/1 -> Nonlinear FK Force Variant Subsystem/2(Displacement), Linear Wave Excitation Force Variant Subsystem/2(Displacement)
  Product/1 -> F_Excitation/1  "F_Excitation"
  Add/1 -> Product/2  "F_wave"
  Switch/1 -> Product/1  "R"

== system GBM1_2022b/Flex Body/Hydrostatic Restoring Force Calculation/Hydrostatic Restoring Force Calculation/Linear and Nonlinear Restoring Force Variant Subsystem ==
  note: If simu.nlHydro == 0, use the linear force option.
      | If simu.nlHydro > 0, use the nonlinear force option.
  note: 1) Add Subsystem or Model blocks as valid variant choices.
      | 2) You cannot connect blocks at this level. At simulation, connectivity is automatically
      | determined, based on the active variant and port name matching.
  In1 : Inport
  In2 : Inport  Port=2
  Linear Hydrostatic Restoring Force : Subsystem  VariantControl=sv_b1_linearHydro
  Nonlinear Hydrostatic Restoring Force : Subsystem  VariantControl=sv_b1_nonlinearHydro
  Out1 : Outport

== system GBM1_2022b/Flex Body/Morrison Element and Viscous Damping Force Calculation/Morison Element and Viscous Damping Force Calculation/Morison Element Variant Subsystem ==
  note: 1) Add Subsystem or Model blocks as valid variant choices.
      | 2) You cannot connect blocks at this level. At simulation, connectivity is automatically
      | determined, based on the active variant and port name matching.
  note: If body.morisonElement.option == 0, Morison element is off and the Morison force is 0
      | If body.morisonElement.option == 1 | 2, Morison element is on
  displacement : Inport
  velocity : Inport  Port=2
  acceleration : Inport  Port=3
  time : Inport  Port=4
  Morison Element Off : Subsystem  VariantControl=sv_b1_MEOff
  Morison Element On : Subsystem  Variant=on  VariantControl=sv_b1_MEOn
  morison_force : Outport

== system GBM1_2022b/Flex Body/Wave Diffraction and Excitation Force Calculation/Wave Diffraction and Excitation Force Calculation/Linear Wave Excitation Force Variant Subsystem ==
  note: 1) Add Subsystem or Model blocks as valid variant choices.
      | 2) You cannot connect blocks at this level. At simulation, connectivity is automatically
      | determined, based on the active variant and port name matching.
  note: No wave includes wave.type == 'noWave' or 'noWaveCIC'
      | Regular wave includes wave.type == 'regular' or 'regularCIC'
      | Irregular wave includes wave.type == 'irregular' or 'spectrumImport'
  Time : Inport
  Displacement : Inport  Port=2
  Irregular Wave Excitation Force : Subsystem  VariantControl=sv_irregularWaves_b1
  Irregular Wave NonLinearYaw : Subsystem  VariantControl=sv_irregularWavesYaw_b1
  No Wave Excitation Force : Subsystem  VariantControl=sv_noWave
  Regular Wave Excitation Force : Subsystem  VariantControl=sv_regularWaves_b1
  Regular Wave NonLinear Yaw : Subsystem  VariantControl=sv_regularWavesYaw_b1
  User Defined Wave Excitation Force : Subsystem  VariantControl=sv_udfWaves
  Linear Excitation : Outport

== system GBM1_2022b/Flex Body/Wave Diffraction and Excitation Force Calculation/Wave Diffraction and Excitation Force Calculation/Nonlinear FK Force Variant Subsystem ==
  note: 1) Add Subsystem or Model blocks as valid variant choices.
      | 2) You cannot connect blocks at this level. At simulation, connectivity is automatically
      | determined, based on the active variant and port name matching.
  note: If simu.nlHydro == 0, use No Nonlinear FroudeKrylov force option (nonlinear force is zero),
      | If simu.nlHydro > 0, use the Nonlinear FroudeKrylov force option,
  Time : Inport
  Displacement : Inport  Port=2
  WaveElv : Inport  Port=3
  No Nonlinear FroudeKrylov Force : Subsystem  VariantControl=sv_b1_linearHydro
  With Nonlinear FroudeKrylov Force : Subsystem  TreatAsAtomicUnit=on  SystemSampleTime=simu.nonlinearDt  VariantControl=sv_b1_nonlinearHydro
  Nonlinear Excitation : Outport

== system GBM1_2022b/Flex Body/Wave Diffraction and Excitation Force Calculation/Wave Diffraction and Excitation Force Calculation/Ramp function ==
  note: The ramp function R, is a smooth function:
      | R = (sin(3*pi/2 + pi * t/Tr) + 1)/2 from t=0 to t=Tr
  Time : Inport
  Add1 : Sum
  Add2 : Sum
  Constant1 : Constant  Value=1/2
  Constant2 : Constant
  Constant3 : Constant  Value=3*pi/2
  Constant4 : Constant  Value=pi
  Divide : Product  Inputs=*/
  Product1 : Product
  Product2 : Product
  Ramp Time : Constant  Value=simu.rampTime
  Sine Wave Function : Sin  TimeSource=Use external signal  SampleTime=0
  R : Outport
  wires:
  Constant1/1 -> Product1/2
  Sine Wave Function/1 -> Add1/2
  Time/1 -> Product2/1
  Product2/1 -> Add2/1
  Add2/1 -> Sine Wave Function/1
  Constant4/1 -> Divide/1
  Add1/1 -> Product1/1
  Divide/1 -> Product2/2  "frequency"
  Ramp Time/1 -> Divide/2  "t_ramp"
  Constant3/1 -> Add2/2  "phase"
  Constant2/1 -> Add1/1
  Product1/1 -> R/1

== system GBM1_2022b/Flex Body/Hydrostatic Restoring Force Calculation/Hydrostatic Restoring Force Calculation/Linear and Nonlinear Restoring Force Variant Subsystem/Linear Hydrostatic Restoring Force ==
  note: The total hydrostatic restoring force is due to a linear stiffness, the vertical buoyancy force (gravity - buoyancy) and a rotational buoyancy force if the center of gravity is not aligned with the center of buoyancy.
      |
      | F_restoring = F_linearRestoringStiffness + F_NetBuoyancy
      |
      | F_linear restoring = hydrostatic restoring coefficient * displacement
      | F_NetBuoyancy = F_gravity - F_buoyancy + F_rotational_buoyancy
      |
      | F_rotational_buoyancy = (cb-cg) x F_buoyancy
      | F_buoyancy = rho*g*V_0
      | F_gravity = m*g
  In1 : Inport
  Add : Sum
  Body Mass : Constant  Value=body.hydroForce.storage.mass
  Linear Restoring Coefficient Matrix : Constant  Value=body.hydroForce.linearHydroRestCoef
  Net Buoyancy Force : Subsystem
  Product2 : Product  Multiplication=Matrix(*)
  Out1 : Outport
  wires:
  Product2/1 -> Add/2  "Linear Restoring Force"
  In1/1 -> Product2/2  "x"
  Linear Restoring Coefficient Matrix/1 -> Product2/1  "K"
  Add/1 -> Out1/1  "F_Restoring"
  Net Buoyancy Force/1(F_NetBuoyancy) -> Add/1  "Net buoyancy force"
  Body Mass/1 -> Net Buoyancy Force/1(Body Mass)  "m"

== system GBM1_2022b/Flex Body/Hydrostatic Restoring Force Calculation/Hydrostatic Restoring Force Calculation/Linear and Nonlinear Restoring Force Variant Subsystem/Nonlinear Hydrostatic Restoring Force ==
  In1 : Inport
  In2 : Inport  Port=2
  Body Mass : Constant  Value=body.hydroForce.storage.mass
  Center of Gravity : Constant  Value=body.centerGravity
  Gravity : Constant  Value=simu.gravity
  Rate Transition : RateTransition
  Rate Transition1 : RateTransition
  Restoring Forces : MATLAB Function  TreatAsAtomicUnit=on  SystemSampleTime=simu.nonlinearDt
  STL areas : Constant  Value=body.geometry.area
  STL centers : Constant  Value=body.geometry.center
  STL normal vectors : Constant  Value=body.geometry.norm
  To Workspace1 : ToWorkspace  VariableName=body1_hspressure_out  SaveFormat=Structure With Time  SampleTime=-1
      settings: Decimation=round(simu.dtOut/simu.dt,0)
  Water Density : Constant  Value=simu.rho
  Out1 : Outport
  wires:
  In1/1 -> Restoring Forces/1(x)
  Center of Gravity/1 -> Restoring Forces/8(cg)
  Gravity/1 -> Restoring Forces/7(g)  "g"
  Water Density/1 -> Restoring Forces/6(rho)
  STL normal vectors/1 -> Restoring Forces/4(tnorm)
  STL centers/1 -> Restoring Forces/3(center)
  In2/1 -> Restoring Forces/2(elv)
  STL areas/1 -> Restoring Forces/5(area)
  Body Mass/1 -> Restoring Forces/9(mass)
  Restoring Forces/2(p) -> Rate Transition1/1
  Rate Transition1/1 -> To Workspace1/1
  Restoring Forces/1(f) -> Rate Transition/1
  Rate Transition/1 -> Out1/1

== system GBM1_2022b/Flex Body/Morrison Element and Viscous Damping Force Calculation/Morison Element and Viscous Damping Force Calculation/Morison Element Variant Subsystem/Morison Element Off ==
  Constant : Constant  Value=zeros(1,body.dof)
  morison_force : Outport
  wires:
  Constant/1 -> morison_force/1

== system GBM1_2022b/Flex Body/Morrison Element and Viscous Damping Force Calculation/Morison Element and Viscous Damping Force Calculation/Morison Element Variant Subsystem/Morison Element On ==
  note: 1) Add Subsystem or Model blocks as valid variant choices.
      | 2) You cannot connect blocks at this level. At simulation, connectivity is automatically
      | determined, based on the active variant and port name matching.
  note: Chooses the appropriate Morison element variant dependent on the wave type. Note that if passive yaw is used, no block is chosen.
      |
      | If wave.type == 'noWave' | 'noWaveCIC' use No Wave Morison element
      | If wave.type == 'regularWave' | 'regularWaveCIC' use Regular Wave Morison element
      | If wave.type == 'irregularWave' or 'spectrumImport' use Irregular Wave Morison element
  displacement : Inport
  velocity : Inport  Port=2
  acceleration : Inport  Port=3
  time : Inport  Port=4
  Irregular Wave Morison Force : Subsystem  TreatAsAtomicUnit=on  SystemSampleTime=simu.morisonDt  VariantControl=sv_irregularWaves_b1
  No Wave Morison Force : Subsystem  VariantControl=sv_noWave
  Regular Wave Morison Force : Subsystem  TreatAsAtomicUnit=on  SystemSampleTime=simu.morisonDt  VariantControl=sv_regularWaves_b1
  morison_force : Outport

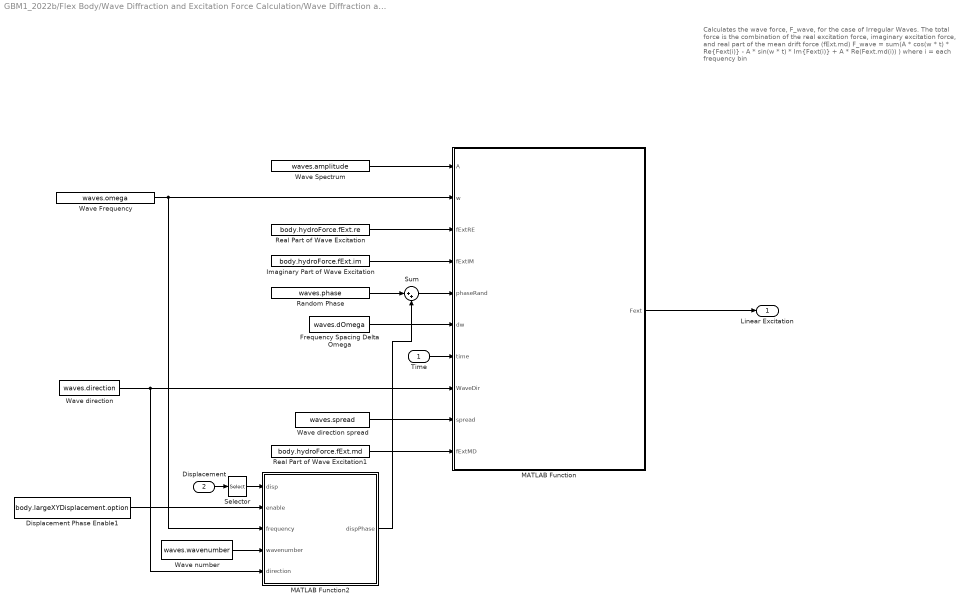
== system GBM1_2022b/Flex Body/Wave Diffraction and Excitation Force Calculation/Wave Diffraction and Excitation Force Calculation/Linear Wave Excitation Force Variant Subsystem/Irregular Wave Excitation Force ==
  note: Calculates the wave force, F_wave, for the case of Irregular Waves.
      |
      | The total force is the combination of the real excitation force, imaginary excitation force, and real part of the mean drift force (fExt.md)
      |
      | F_wave =   sum(A * cos(w * t) * Re{Fext(i)}
      |                            -  A * sin(w * t) * Im{Fext(i)}
      |                            + A * Re(Fext.md(i))
      |                            )
      |
      | where i = each frequency bin
  Time : Inport
  Displacement : Inport  Port=2
  Displacement Phase Enable1 : Constant  Value=body.largeXYDisplacement.option
  Frequency Spacing Delta Omega : Constant  Value=waves.dOmega  VectorParams1D=off
  Imaginary Part of Wave Excitation : Constant  Value=body.hydroForce.fExt.im  VectorParams1D=off
  MATLAB Function : MATLAB Function  TreatAsAtomicUnit=on
  MATLAB Function2 : MATLAB Function  TreatAsAtomicUnit=on
  Random Phase : Constant  Value=waves.phase  VectorParams1D=off
  Real Part of Wave Excitation : Constant  Value=body.hydroForce.fExt.re  VectorParams1D=off
  Real Part of Wave Excitation1 : Constant  Value=body.hydroForce.fExt.md  VectorParams1D=off
  Selector : Selector  IndexOptions=Index vector (dialog)  Indices=[1 2]  OutputSizes=1
  Sum : Sum  Inputs=|++
  Wave Frequency : Constant  Value=waves.omega  VectorParams1D=off
  Wave Spectrum : Constant  Value=waves.amplitude  VectorParams1D=off
  Wave direction : Constant  Value=waves.direction  VectorParams1D=off
  Wave direction spread : Constant  Value=waves.spread  VectorParams1D=off
  Wave number : Constant  Value=waves.wavenumber  VectorParams1D=off
  Linear Excitation : Outport
  wires:
  Selector/1 -> MATLAB Function2/1(disp)
  Wave number/1 -> MATLAB Function2/4(wavenumber)
  Displacement Phase Enable1/1 -> MATLAB Function2/2(enable)
  Displacement/1 -> Selector/1
  MATLAB Function2/1(dispPhase) -> Sum/2
  Sum/1 -> MATLAB Function/5(phaseRand)
  Random Phase/1 -> Sum/1
  Real Part of Wave Excitation1/1 -> MATLAB Function/10(fExtMD)
  Wave direction/1 -> MATLAB Function/8(WaveDir), MATLAB Function2/5(direction)
  Wave direction spread/1 -> MATLAB Function/9(spread)
  Frequency Spacing Delta Omega/1 -> MATLAB Function/6(dw)
  Time/1 -> MATLAB Function/7(time)
  Wave Spectrum/1 -> MATLAB Function/1(A)
  Real Part of Wave Excitation/1 -> MATLAB Function/3(fExtRE)
  Imaginary Part of Wave Excitation/1 -> MATLAB Function/4(fExtIM)
  Wave Frequency/1 -> MATLAB Function/2(w), MATLAB Function2/3(frequency)
  MATLAB Function/1(Fext) -> Linear Excitation/1
